simulink model "prob2"  (R2020a)
settings: Solver=VariableStepAuto  StartTime=0.0  StopTime=100  MaxStep=0.01  RelTol=1e-3
values from neighbouring files (symbols this model uses):
  b = 350.0    [data.sldd]    (also in para.m = 350)
  k1 = 80000.0    [data.sldd]    (also in para.m = 80000)
  k2 = 500000.0    [data.sldd]    (also in para.m = 500000)
  m1 = 2500.0    [data.sldd]    (also in para.m = 2500)
  m2 = 320.0    [data.sldd]    (also in para.m = 320)
settings Model: DataDictionary=data.sldd  Creator=vijay  LastModifiedBy=vijay

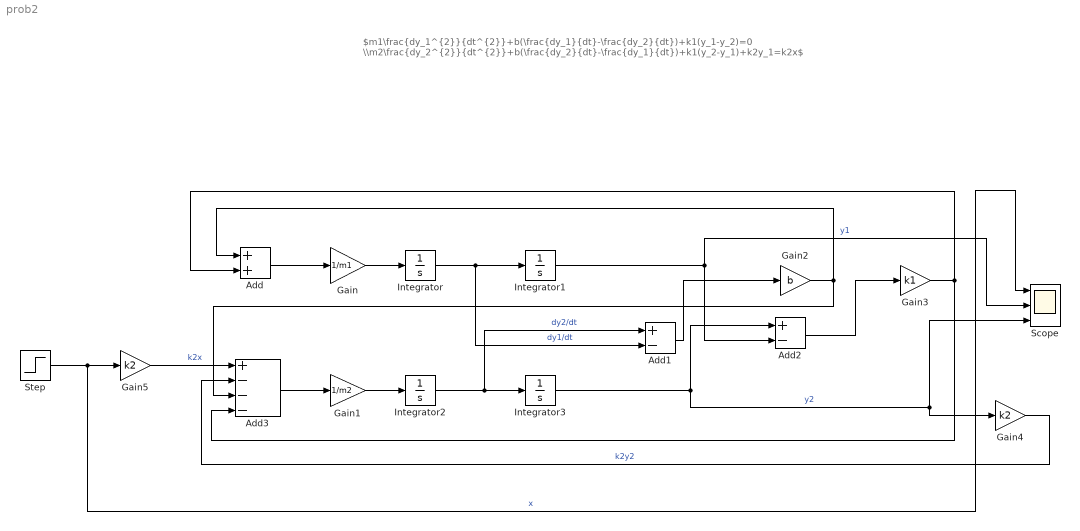
== system prob2 ==
  note: $m1\frac{dy_1^{2}}{dt^{2}}+b(\frac{dy_1}{dt}-\frac{dy_2}{dt})+k1(y_1-y_2)=0 \\m2\frac{dy_2^{2}}{dt^{2}}+b(\frac{dy_2}{dt}-\frac{dy_1}{dt})+k1(y_2-y_1)+k2y_1=k2x$
  Add : Sum
  Add1 : Sum  Inputs=+-
  Add2 : Sum  Inputs=+-
  Add3 : Sum  Inputs=+---
  Gain : Gain  Gain=1/m1
  Gain1 : Gain  Gain=1/m2
  Gain2 : Gain  Gain=b
  Gain3 : Gain  Gain=k1
  Gain4 : Gain  Gain=k2
  Gain5 : Gain  Gain=k2
  Integrator{,1..3} (4 alike) : Integrator
  Scope : Scope  NumInputPorts=3
  Step : Step  Time=5  SampleTime=0
  wires:
  Integrator/1 -> Add1/2, Integrator1/1  "dy1/dt"
  Integrator2/1 -> Add1/1, Integrator3/1  "dy2/dt"
  Gain/1 -> Integrator/1
  Gain1/1 -> Integrator2/1
  Integrator3/1 -> Scope/3, Gain4/1, Add2/1  "y2"
  Integrator1/1 -> Add2/2, Scope/2  "y1"
  Add1/1 -> Gain2/1
  Add2/1 -> Gain3/1
  Add/1 -> Gain/1
  Gain2/1 -> Add3/3, Add/1
  Gain3/1 -> Add/2, Add3/4
  Add3/1 -> Gain1/1
  Gain4/1 -> Add3/2  "k2y2"
  Gain5/1 -> Add3/1  "k2x"
  Step/1 -> Scope/1, Gain5/1  "x"
